simulink model "right"  (R2016b)
settings: Solver=VariableStepAuto  StartTime=0.0  StopTime=10.0  RelTol=1e-3
libraries: TLMLib x1
settings Model: Creator=robbr48  LastModifiedBy=robbr48

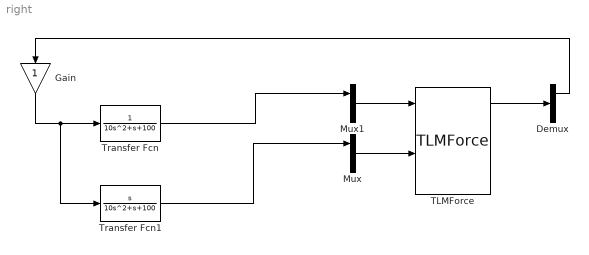
== system right ==
  Demux : Demux  Outputs=3
  Gain : Gain
  Mux : Mux  Inputs=3
  Mux1 : Mux  Inputs=3
  TLMForce : TLMLib/TLMForce
  Transfer Fcn : TransferFcn  Denominator=[10 1 100]
  Transfer Fcn1 : TransferFcn  Numerator=[1 0]  Denominator=[10 1 100]
  wires:
  TLMForce/1 -> Demux/1
  Mux/1 -> TLMForce/3
  Mux1/1 -> TLMForce/1
  Gain/1 -> Transfer Fcn1/1, Transfer Fcn/1
  Transfer Fcn1/1 -> Mux/1
  Transfer Fcn/1 -> Mux1/1
  Demux/1 -> Gain/1
